simulink model "pendule_inv_capteur_etu"  (R2017a)
settings: Solver=VariableStepAuto  StartTime=0.0  StopTime=tf  RelTol=1e-3
values from neighbouring files (symbols this model uses):
  K = [30 10]    [exemple_test_pendule_inv.m]    (also in exemple_test_pendule_inv_capteur.m = [10 1]; exemple_test_pendule_inv_echant.m)
  x0 = [pi/10 0]    [exemple_test_pendule_inv.m]    (also in exemple_test_pendule_inv_capteur.m = [pi/20 0]; exemple_test_pendule_inv_echant.m = [pi/20 0])
settings Model: Creator=mkerrand  LastModifiedBy=mlarzul

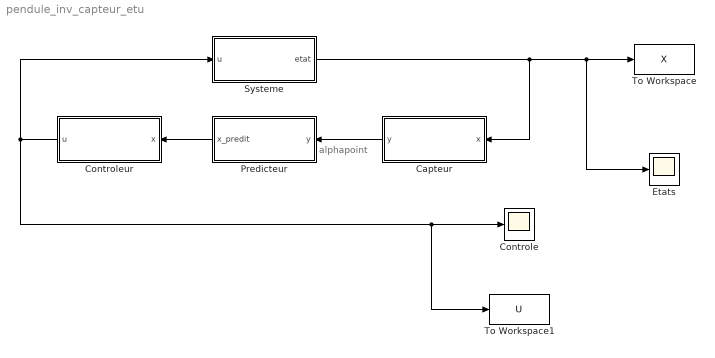
== system pendule_inv_capteur_etu ==
  note: alphapoint
  Capteur : Subsystem
  Controle : Scope
  Controleur : Subsystem
  Etats : Scope
  Predicteur : Subsystem
  Systeme : Subsystem
  To Workspace : ToWorkspace  VariableName=X  SaveFormat=Timeseries  SampleTime=-1
  To Workspace1 : ToWorkspace  VariableName=U  SaveFormat=Timeseries  SampleTime=-1
  wires:
  Systeme/1("etat ") -> Capteur/1(x), Etats/1, To Workspace/1
  Controleur/1(u) -> Controle/1, To Workspace1/1, Systeme/1(u)
  Predicteur/1("x_predit ") -> Controleur/1(x)
  Capteur/1("y ") -> Predicteur/1(y)

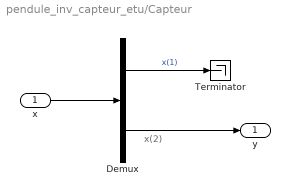
== system pendule_inv_capteur_etu/Capteur ==
  note: x(2)
  x : Inport
  Demux : Demux  Outputs=2
  Terminator : Terminator
  "y " : Outport
  wires:
  x/1 -> Demux/1
  Demux/2 -> "y "/1
  Demux/1 -> Terminator/1  "x(1)"

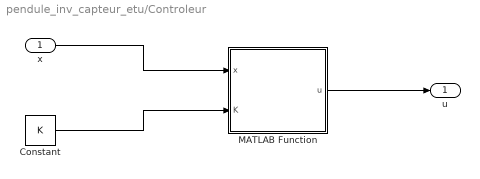
== system pendule_inv_capteur_etu/Controleur ==
  x : Inport
  Constant : Constant  Value=K
  MATLAB Function : MATLAB Function  TreatAsAtomicUnit=on
  u : Outport
  wires:
  MATLAB Function/1(u) -> u/1
  x/1 -> MATLAB Function/1(x)
  Constant/1 -> MATLAB Function/2(K)

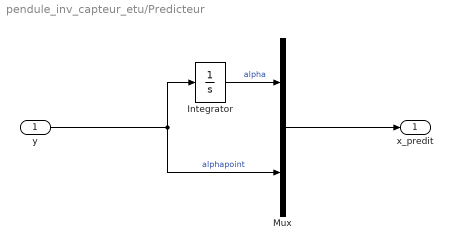
== system pendule_inv_capteur_etu/Predicteur ==
  y : Inport
  Integrator : Integrator  InitialCondition=x0(1)
  Mux : Mux  Inputs=2
  "x_predit " : Outport
  wires:
  y/1 -> Mux/2, Integrator/1  "alphapoint"
  Mux/1 -> "x_predit "/1
  Integrator/1 -> Mux/1  "alpha"

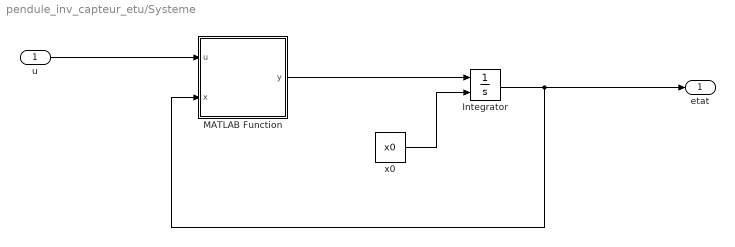
== system pendule_inv_capteur_etu/Systeme ==
  u : Inport
  Integrator : Integrator  InitialConditionSource=external
  MATLAB Function : MATLAB Function  TreatAsAtomicUnit=on
  x0 : Constant  Value=x0
  "etat " : Outport
  wires:
  u/1 -> MATLAB Function/1(u)
  MATLAB Function/1(y) -> Integrator/1
  Integrator/1 -> "etat "/1, MATLAB Function/2(x)
  x0/1 -> Integrator/2

== matlab function pendule_inv_capteur_etu/Systeme/MATLAB Function ==
  data: u input; y output; x input
function y = fcn(u,x)
    g=9.81;
    l=10;
    
    y1 = x(2);
    y2 = g/l*sin(x(1)) - (cos(x(1))*u)/l;
    y=[y1 y2]';

== matlab function pendule_inv_capteur_etu/Controleur/MATLAB Function ==
  data: x input; u output; K input
function u = fcn(x,K)
    
    xe = [0 0];
    ue = 0;
    
    u = ue + K'*(x-xe') ;
